simulink model "Lab3_jinjin"  (R2022a)
settings: Solver=VariableStepAuto  StartTime=0.0  StopTime=10  RelTol=1e-3
libraries: sharedutil x2
settings Model: Creator=이진진  LastModifiedBy=이진진
settings DebuggingCC: UnconnectedInputMsg=warning  UnconnectedOutputMsg=warning  UnconnectedLineMsg=warning
settings RTWCC: DLArmComputeVersion=19.05

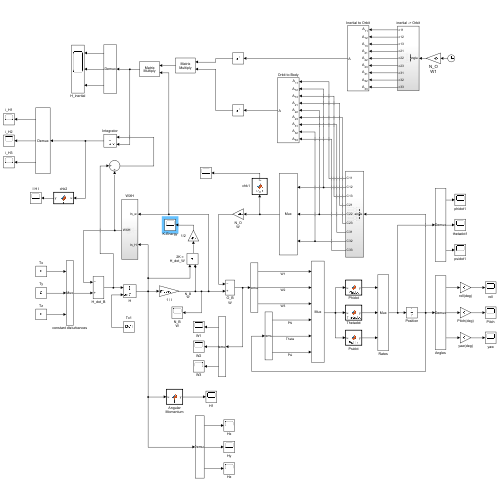
[thumbnail: Simulink's stored preview of the top-level diagram]
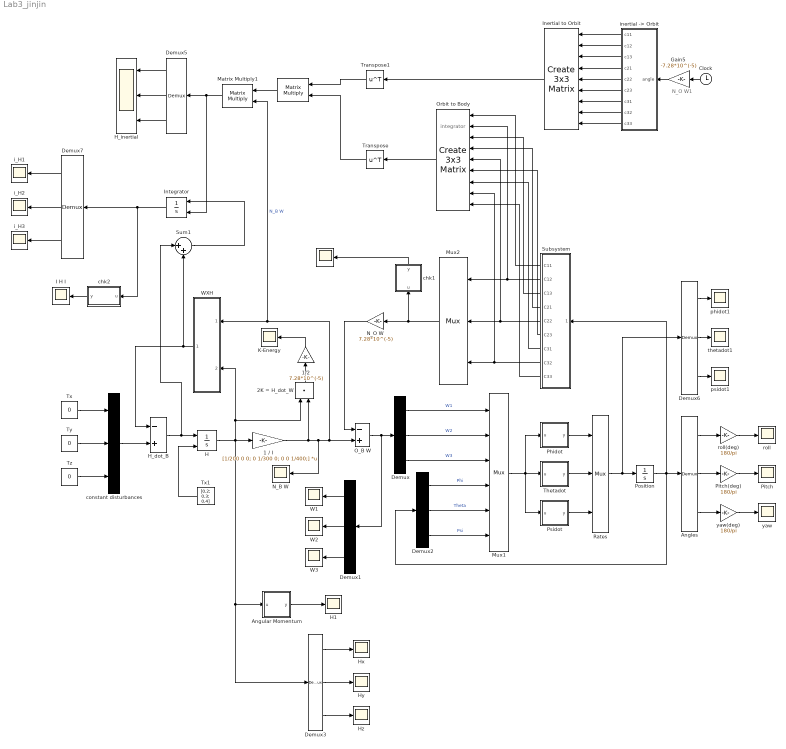
== system Lab3_jinjin ==
  note: N_O
      | W1
  note: integrator
  " " : Scope
  "  " : Product  Multiplication=Matrix(*)
  1 / I : Gain  Gain=[1/200 0 0; 0 1/300 0; 0 0 1/400;]  Multiplication=Matrix(K*u) (u vector)
  1/2 : Gain  Gain=7.28*10^(-5)
  2K = H_dot_W : DotProduct  OutDataTypeStr=Inherit: Inherit via internal rule
  Angles : Demux  Outputs=3
      settings: DisplayOption=none
  Angular Momentum : MATLAB Function  TreatAsAtomicUnit=on
  Clock : Clock
  Demux{,1..3,5..7} (7 alike) : Demux  Outputs=3
      settings: DisplayOption=none
  Gain5 : Gain  Gain=-7.28*10^(-5)
  H : Integrator  InitialConditionSource=external  InitialCondition=[0.2 0.3 0.4]
  H1 : Scope
  H_dot_B : Sum  Inputs=-+
  H_inertial : Scope  NumInputPorts=3
  Hx : Scope
  Hy : Scope
  Hz : Scope
  I H I : Scope
  Inertial to Orbit : sharedutil/Create 3x3 Matrix  aMode=aMode
      settings: SourceProductBaseCode=AE,PW,DR,MT,VE
  Integrator : Integrator  InitialConditionSource=external
  K-Energy : Scope
  Matrix Multiply1 : Product  Multiplication=Matrix(*)
  Mux1 : Mux  Inputs=6
  Mux2 : Mux  Inputs=3
  N_B W : Scope
  N_O W : Gain  Gain=7.28*10^(-5)
  O_B W : Sum  Inputs=-+
  Orbit to Body : sharedutil/Create 3x3 Matrix  aMode=aMode
      settings: SourceProductBaseCode=AE,PW,DR,MT,VE
  Phidot : MATLAB Function  TreatAsAtomicUnit=on
  Pitch : Scope
  Pitch(deg) : Gain  Gain=180/pi
  Position : Integrator  InitialCondition=[10*pi/180, 20*pi/180, 30*pi/180]
  Psidot : MATLAB Function  TreatAsAtomicUnit=on
  Rates : Mux  Inputs=3
  Subsystem : Subsystem
  Sum1 : Sum  Inputs=|++
  Thetadot : MATLAB Function  TreatAsAtomicUnit=on
  Transpose : Math  Operator=transpose
  Transpose1 : Math  Operator=transpose
  Tx : Constant  Value=0
  Tx1 : Constant  Value=[0.2; 0.3; 0.4]
  Ty : Constant  Value=0
  Tz : Constant  Value=0
  W1 : Scope
  W2 : Scope
  W3 : Scope
  WXH : Subsystem
  chk1 : MATLAB Function  TreatAsAtomicUnit=on
  chk2 : MATLAB Function  TreatAsAtomicUnit=on
  constant disturbances : Mux  Inputs=3
  i_H1 : Scope
  i_H2 : Scope
  i_H3 : Scope
  "inertial -> Orbit" : Subsystem
  phidot1 : Scope
  psidot1 : Scope
  roll : Scope
  roll(deg) : Gain  Gain=180/pi
  thetadot1 : Scope
  yaw : Scope
  yaw(deg) : Gain  Gain=180/pi
  wires:
  Demux/1 -> Mux1/1  "W1"
  Demux/2 -> Mux1/2  "W2"
  Demux/3 -> Mux1/3  "W3"
  Demux1/1 -> W1/1
  Demux1/2 -> W2/1
  Demux1/3 -> W3/1
  Demux2/1 -> Mux1/4  "Phi"
  Demux2/2 -> Mux1/5  "Theta"
  Demux2/3 -> Mux1/6  "Psi"
  Tx/1 -> constant disturbances/1
  Ty/1 -> constant disturbances/2
  Tz/1 -> constant disturbances/3
  O_B W/1 -> Demux1/1, Demux/1
  Mux1/1 -> Thetadot/1(u), Psidot/1(u), Phidot/1(u)
  Phidot/1(y) -> Rates/1
  Thetadot/1(y) -> Rates/2
  Psidot/1(y) -> Rates/3
  Rates/1 -> Position/1, Demux6/1
  Position/1 -> Demux2/1, Subsystem/1(angle), Angles/1
  Angles/1 -> roll(deg)/1
  Angles/2 -> Pitch(deg)/1
  Angles/3 -> yaw(deg)/1
  roll(deg)/1 -> roll/1
  Pitch(deg)/1 -> Pitch/1
  yaw(deg)/1 -> yaw/1
  Subsystem/2(C12) -> Mux2/1, Orbit to Body/2
  Subsystem/5(C22) -> Orbit to Body/5, Mux2/2
  Subsystem/8(C32) -> Orbit to Body/8, Mux2/3
  Mux2/1 -> chk1/1(u), N_O W/1
  N_O W/1 -> O_B W/1
  chk1/1(y) -> " "/1
  constant disturbances/1 -> H_dot_B/2
  H/1 -> Angular Momentum/1(u), Demux3/1, 1 / I/1, 2K = H_dot_W/1, WXH/2(In_H)
  Tx1/1 -> H/2
  1 / I/1 -> N_B W/1, O_B W/2, WXH/1(In_w), Matrix Multiply1/2, 2K = H_dot_W/2  "N_B W"
  Demux6/1 -> phidot1/1
  Demux6/2 -> thetadot1/1
  Demux6/3 -> psidot1/1
  2K = H_dot_W/1 -> 1/2/1
  1/2/1 -> K-Energy/1
  Demux3/1 -> Hx/1
  Demux3/2 -> Hy/1
  Demux3/3 -> Hz/1
  Angular Momentum/1(y) -> H1/1
  Clock/1 -> Gain5/1
  Gain5/1 -> "inertial -> Orbit"/1(angle)
  "inertial -> Orbit"/5(c22) -> Inertial to Orbit/5
  "inertial -> Orbit"/6(c23) -> Inertial to Orbit/6
  "inertial -> Orbit"/7(c31) -> Inertial to Orbit/7
  "inertial -> Orbit"/8(c32) -> Inertial to Orbit/8
  "inertial -> Orbit"/9(c33) -> Inertial to Orbit/9
  "inertial -> Orbit"/4(c21) -> Inertial to Orbit/4
  "inertial -> Orbit"/3(c13) -> Inertial to Orbit/3
  Subsystem/1(C11) -> Orbit to Body/1
  Subsystem/3(C13) -> Orbit to Body/3
  Subsystem/4(C21) -> Orbit to Body/4
  Subsystem/6(C23) -> Orbit to Body/6
  Subsystem/7(C31) -> Orbit to Body/7
  Subsystem/9(C33) -> Orbit to Body/9
  Inertial to Orbit/1 -> Transpose1/1
  Orbit to Body/1 -> Transpose/1
  Transpose/1 -> "  "/2
  Transpose1/1 -> "  "/1
  "  "/1 -> Matrix Multiply1/1
  Demux5/2 -> H_inertial/2
  Demux5/1 -> H_inertial/1
  Demux5/3 -> H_inertial/3
  Matrix Multiply1/1 -> Integrator/2, Demux5/1
  WXH/1(WXH) -> Sum1/2, H_dot_B/1
  Sum1/1 -> Integrator/1
  chk2/1(y) -> I H I/1
  Demux7/2 -> i_H2/1
  H_dot_B/1 -> Sum1/1, H/1
  Integrator/1 -> chk2/1(u), Demux7/1
  Demux7/1 -> i_H1/1
  Demux7/3 -> i_H3/1
  "inertial -> Orbit"/1(c11) -> Inertial to Orbit/1
  "inertial -> Orbit"/2(c12) -> Inertial to Orbit/2

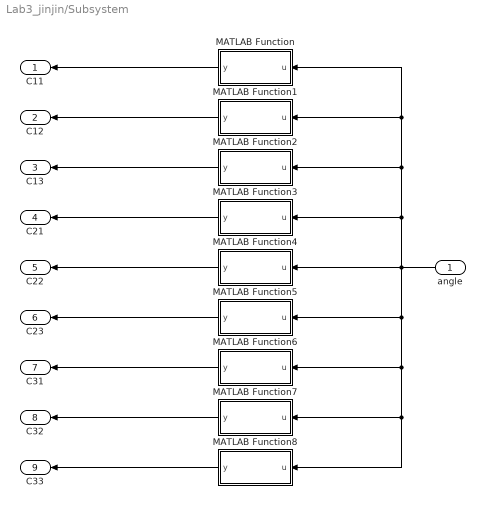
== system Lab3_jinjin/Subsystem ==
  angle : Inport
  MATLAB Function : MATLAB Function  TreatAsAtomicUnit=on
  MATLAB Function1 : MATLAB Function  TreatAsAtomicUnit=on
  MATLAB Function2 : MATLAB Function  TreatAsAtomicUnit=on
  MATLAB Function3 : MATLAB Function  TreatAsAtomicUnit=on
  MATLAB Function4 : MATLAB Function  TreatAsAtomicUnit=on
  MATLAB Function5 : MATLAB Function  TreatAsAtomicUnit=on
  MATLAB Function6 : MATLAB Function  TreatAsAtomicUnit=on
  MATLAB Function7 : MATLAB Function  TreatAsAtomicUnit=on
  MATLAB Function8 : MATLAB Function  TreatAsAtomicUnit=on
  C11 : Outport
  C12 : Outport  Port=2
  C13 : Outport  Port=3
  C21 : Outport  Port=4
  C22 : Outport  Port=5
  C23 : Outport  Port=6
  C31 : Outport  Port=7
  C32 : Outport  Port=8
  C33 : Outport  Port=9
  wires:
  MATLAB Function8/1(y) -> C33/1
  MATLAB Function7/1(y) -> C32/1
  MATLAB Function6/1(y) -> C31/1
  MATLAB Function5/1(y) -> C23/1
  MATLAB Function4/1(y) -> C22/1
  MATLAB Function3/1(y) -> C21/1
  MATLAB Function2/1(y) -> C13/1
  MATLAB Function1/1(y) -> C12/1
  MATLAB Function/1(y) -> C11/1
  angle/1 -> MATLAB Function/1(u), MATLAB Function1/1(u), MATLAB Function2/1(u), MATLAB Function3/1(u), MATLAB Function4/1(u), MATLAB Function5/1(u), MATLAB Function6/1(u), MATLAB Function7/1(u), MATLAB Function8/1(u)

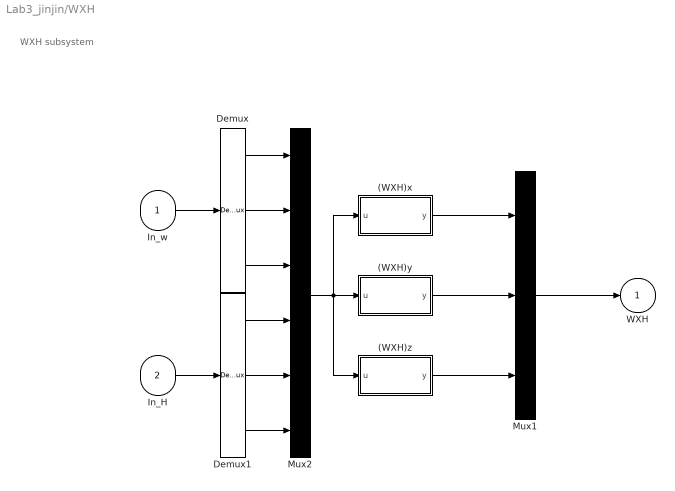
== system Lab3_jinjin/WXH ==
  note: WXH subsystem
  In_w : Inport
  In_H : Inport  Port=2
  (WXH)x : MATLAB Function  TreatAsAtomicUnit=on
  (WXH)y : MATLAB Function  TreatAsAtomicUnit=on
  (WXH)z : MATLAB Function  TreatAsAtomicUnit=on
  Demux : Demux  Outputs=3
      settings: DisplayOption=none
  Demux1 : Demux  Outputs=3
      settings: DisplayOption=none
  Mux1 : Mux  Inputs=3
  Mux2 : Mux  Inputs=6
  WXH : Outport
  wires:
  (WXH)x/1(y) -> Mux1/1
  Mux2/1 -> (WXH)z/1(u), (WXH)y/1(u), (WXH)x/1(u)
  Mux1/1 -> WXH/1
  In_H/1 -> Demux1/1
  Demux1/3 -> Mux2/6
  Demux1/2 -> Mux2/5
  Demux1/1 -> Mux2/4
  Demux/3 -> Mux2/3
  Demux/2 -> Mux2/2
  Demux/1 -> Mux2/1
  In_w/1 -> Demux/1
  (WXH)z/1(y) -> Mux1/3
  (WXH)y/1(y) -> Mux1/2

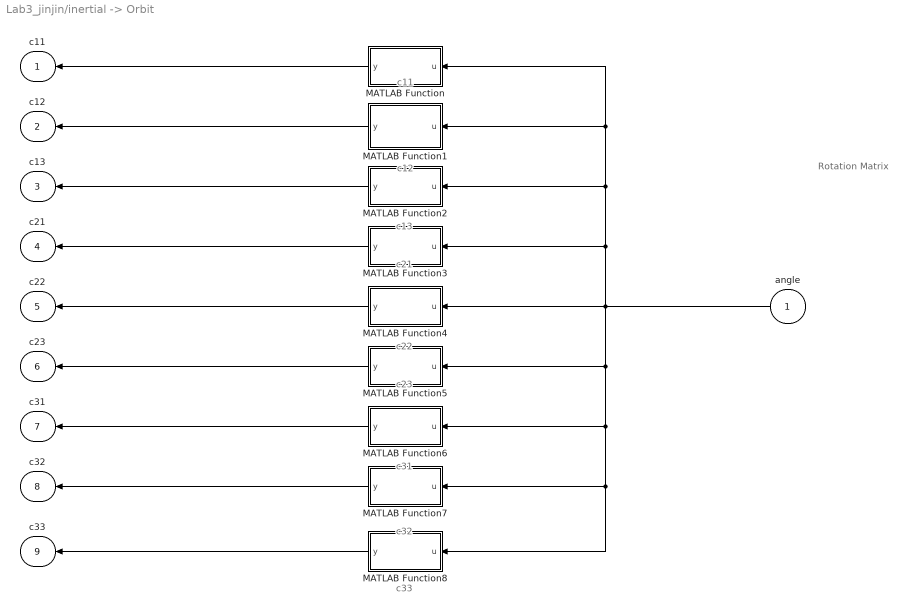
== system Lab3_jinjin/inertial -> Orbit ==
  note: c33
  note: c32
  note: c31
  note: c23
  note: c22
  note: c21
  note: c13
  note: c12
  note: Rotation Matrix
  note: c11
  angle : Inport
  MATLAB Function : MATLAB Function  TreatAsAtomicUnit=on
  MATLAB Function1 : MATLAB Function  TreatAsAtomicUnit=on
  MATLAB Function2 : MATLAB Function  TreatAsAtomicUnit=on
  MATLAB Function3 : MATLAB Function  TreatAsAtomicUnit=on
  MATLAB Function4 : MATLAB Function  TreatAsAtomicUnit=on
  MATLAB Function5 : MATLAB Function  TreatAsAtomicUnit=on
  MATLAB Function6 : MATLAB Function  TreatAsAtomicUnit=on
  MATLAB Function7 : MATLAB Function  TreatAsAtomicUnit=on
  MATLAB Function8 : MATLAB Function  TreatAsAtomicUnit=on
  c11 : Outport
  c12 : Outport  Port=2
  c13 : Outport  Port=3
  c21 : Outport  Port=4
  c22 : Outport  Port=5
  c23 : Outport  Port=6
  c31 : Outport  Port=7
  c32 : Outport  Port=8
  c33 : Outport  Port=9
  wires:
  MATLAB Function8/1(y) -> c33/1
  MATLAB Function7/1(y) -> c32/1
  MATLAB Function6/1(y) -> c31/1
  MATLAB Function5/1(y) -> c23/1
  MATLAB Function4/1(y) -> c22/1
  MATLAB Function3/1(y) -> c21/1
  MATLAB Function2/1(y) -> c13/1
  MATLAB Function1/1(y) -> c12/1
  MATLAB Function/1(y) -> c11/1
  angle/1 -> MATLAB Function2/1(u), MATLAB Function/1(u), MATLAB Function1/1(u), MATLAB Function3/1(u), MATLAB Function4/1(u), MATLAB Function5/1(u), MATLAB Function6/1(u), MATLAB Function7/1(u), MATLAB Function8/1(u)

== matlab function Lab3_jinjin/WXH/(WXH)y ==
  data: u input; y output
function y = fcn(u)

y = u(1)*u(6) - u(3)*u(4);

end

== matlab function Lab3_jinjin/WXH/(WXH)z ==
  data: u input; y output
function y = fcn(u)

y = u(1)*u(5) - u(2)*u(4);

end

== matlab function Lab3_jinjin/Angular Momentum ==
  data: u input; y output
function y = f(u)

y = sqrt(u(1)^2 + u(2)^2 + u(3)^2);

end

== matlab function Lab3_jinjin/inertial -> Orbit/MATLAB Function ==
  data: u input; y output
function y = fcn(u)

y = cos(u(1));

end

== matlab function Lab3_jinjin/inertial -> Orbit/MATLAB Function1 ==
  data: u input; y output
function y = fcn(u)

y = 0;

end

== matlab function Lab3_jinjin/Phidot ==
  data: u input; y output
function y = Phidot(u)

y = u(1) + sin(u(4))*tan(u(5))*u(2) + cos(u(4))*tan(u(5))*u(3);

end

== matlab function Lab3_jinjin/inertial -> Orbit/MATLAB Function2 ==
  data: u input; y output
function y = fcn(u)

y = -sin(u(1));

end

== matlab function Lab3_jinjin/inertial -> Orbit/MATLAB Function3 ==
  data: u input; y output
function y = fcn(u)

y = 0;

end

== matlab function Lab3_jinjin/inertial -> Orbit/MATLAB Function4 ==
  data: u input; y output
function y = fcn(u)

y = 1;

end

== matlab function Lab3_jinjin/inertial -> Orbit/MATLAB Function5 ==
  data: u input; y output
function y = fcn(u)

y = 0;

end

== matlab function Lab3_jinjin/inertial -> Orbit/MATLAB Function6 ==
  data: u input; y output
function y = fcn(u)

y = sin(u(1));

end

== matlab function Lab3_jinjin/inertial -> Orbit/MATLAB Function7 ==
  data: u input; y output
function y = fcn(u)

y = 0;
end

== matlab function Lab3_jinjin/inertial -> Orbit/MATLAB Function8 ==
  data: u input; y output
function y = fcn(u)

y = cos(u(1));

end

== matlab function Lab3_jinjin/chk2 ==
  data: u input; y output
function y = f(u)

y = sqrt((u(1))^2 + (u(2))^2 + (u(3))^2);

end

== matlab function Lab3_jinjin/Psidot ==
  data: u input; y output
function y = Psidot(u)

y = (sin(u(4))/cos(u(5)))*u(2) + (cos(u(4))/cos(u(5))*u(3));

end

== matlab function Lab3_jinjin/Subsystem/MATLAB Function ==
  data: u input; y output
function y = C11(u)

y = cos(u(3))*cos(u(2));

end

== matlab function Lab3_jinjin/Subsystem/MATLAB Function1 ==
  data: u input; y output
function y = C12(u)

y = sin(u(3))*cos(u(2));

end

== matlab function Lab3_jinjin/Subsystem/MATLAB Function2 ==
  data: u input; y output
function y = C13(u)

y = -sin(u(2));

end

== matlab function Lab3_jinjin/Subsystem/MATLAB Function3 ==
  data: u input; y output
function y = C21(u)

y = -sin(u(3))*cos(u(1)) + cos(u(3))*sin(u(2))*sin(u(1));

end

== matlab function Lab3_jinjin/Subsystem/MATLAB Function4 ==
  data: u input; y output
function y = C22(u)

y = cos(u(3))*cos(u(1)) + sin(u(3))*sin(u(2))*sin(u(1));

end

== matlab function Lab3_jinjin/Subsystem/MATLAB Function5 ==
  data: u input; y output
function y = C23(u)

y = cos(u(2))*sin(u(1));

end

== matlab function Lab3_jinjin/Thetadot ==
  data: u input; y output
function y = Thetadot(u)

y = cos(u(4))*u(2) - sin(u(4))*u(3);

end

== matlab function Lab3_jinjin/Subsystem/MATLAB Function6 ==
  data: u input; y output
function y = C31(u)

y = sin(u(3))*sin(u(1)) + cos(u(3))*sin(u(2))*cos(u(1));

end

== matlab function Lab3_jinjin/Subsystem/MATLAB Function7 ==
  data: u input; y output
function y = C32(u)

y = -cos(u(3))*sin(u(1)) + sin(u(3))*sin(u(2))*cos(u(1));

end

== matlab function Lab3_jinjin/Subsystem/MATLAB Function8 ==
  data: u input; y output
function y = C33(u)

y = cos(u(2))*cos(u(1));

end

== matlab function Lab3_jinjin/chk1 ==
  data: u input; y output
function y = chk1(u)

y = sqrt(u(1)^2 + u(2)^2 + u(3)^2) - 1;

end

== matlab function Lab3_jinjin/WXH/(WXH)x ==
  data: u input; y output
function y = fcn(u)

y = u(2)*u(6) - u(3)*u(5);

end
